simulink model "MMS_ESC_K_B_mixed_3"  (R2019b)
settings: Solver=ode4  StartTime=par.sym.TStart  StopTime=par.sym.TStop  FixedStep=par.sym.max_dt  MaxStep=par.sym.max_dt  RelTol=1e-3
undefined symbols (not defined in the file): b, B_0, beta_B, beta_K, eta_B, eta_K, k, K_0, k_B, k_K, lambda_B, lambda_K, m, m1_B0, m1_K0, m2_B0, m2_K0, N_delay, par, Q1_B0, Q1_K0, Q2_B0, Q2_K0, rho_B, rho_K, sigma, T_tran, W_B, W_K, w_wav
libraries: simulink x2
settings Model: Creator=Vitù  LastModifiedBy=User
settings DataIOCC: SaveFormat=Array  SaveOutput=off  SignalLogging=off  DSMLogging=off  ReturnWorkspaceOutputs=off  TimeSaveName=TIME  OutputSaveName=Yout  OutputOption=SpecifiedOutputTimes  OutputTimes=[par.sym.TStart:par.sym.Outputdt:par.sym.TStop]
settings OptimizationCC: ExpressionDepthLimit=2147483647  LifeSpan=inf
settings DebuggingCC: UnderspecifiedInitializationDetection=Classic  MergeDetectMultiDrivingBlocksExec=none  SolverPrmCheckMsg=warning  AllowSymbolicDim=off  StateNameClashWarn=warning  SFUnexpectedBacktrackingDiag=warning  SFNoUnconditionalDefaultTransitionDiag=warning  SFExecutionAtInitializationDiag=none  ArithmeticOperatorsInVariantConditions=warning
settings HardwareCC: ProdBitPerPointer=32  ProdBitPerSizeT=32  ProdBitPerPtrDiffT=32  ProdLargestAtomicFloat=None  ProdIntDivRoundTo=Undefined  ProdEndianess=Unspecified  ProdWordSize=32  ProdHWDeviceType=32-bit Generic
settings ModelReferenceCC: PropagateSignalLabelsOutOfModel=off
settings SFSimCC: SimUseLocalCustomCode=off  CustomCodeUndefinedFunction=UseInterfaceOnly
settings RTWCC: RTWUseLocalCustomCode=off
settings CodeAppCC: StateflowObjectComments=on
settings GRTTargetCC: TargetLangStandard=C89/C90 (ANSI)  GeneratePreprocessorConditionals=Disable all
settings ConfigComp: CovMetricSettings=dw  CovHtmlReporting=on  CovSaveCumulativeToWorkspaceVar=on  CovSaveSingleToWorkspaceVar=on  CovExternalEMLEnable=off  CovSFcnEnable=off
settings SimscapeCC: SimscapeNormalizeSystem=off
settings ConfigurationSet: Description=SimMechanics 2G

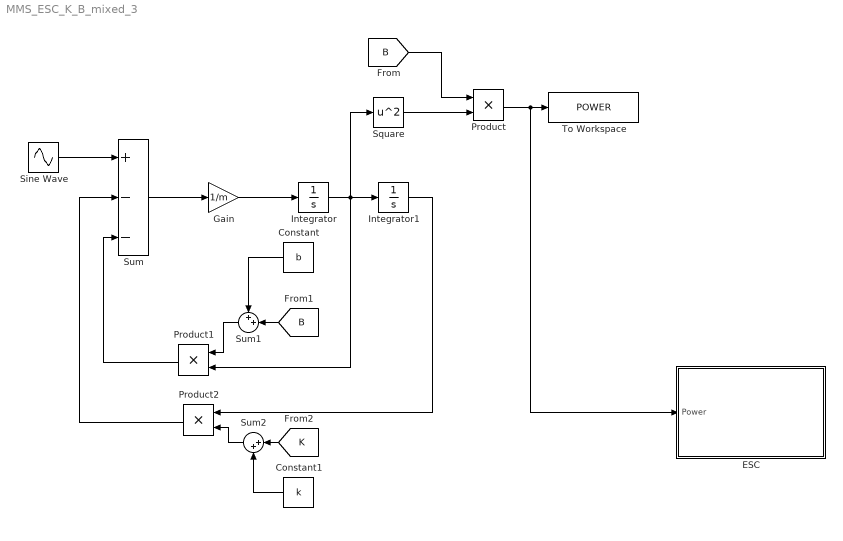
== system MMS_ESC_K_B_mixed_3 ==
  Constant : Constant  Value=b
  Constant1 : Constant  Value=k
  ESC : Subsystem
  Gain : Gain  Gain=1/m
  Integrator : Integrator
  Integrator1 : Integrator
  Product : Product
  Product1 : Product
  Product2 : Product
  Sine Wave : Sin  Amplitude=par.H  Frequency=w_wav  SampleTime=0
  Square : Math  Operator=square  SignedPower=off  SaturateOnIntegerOverflow=on
  Sum : Sum  Inputs=+--
  Sum1 : Sum  Inputs=++|
  Sum2 : Sum  Inputs=|++
  To Workspace : ToWorkspace  VariableName=POWER  SampleTime=-1
  wires:
  Integrator1/1 -> Product2/1
  Product/1 -> ESC/1(Power), To Workspace/1
  Product1/1 -> Sum/3
  Gain/1 -> Integrator/1
  Square/1 -> Product/2
  Sum/1 -> Gain/1
  Integrator/1 -> Product1/2, Square/1, Integrator1/1
  Product2/1 -> Sum/2
  Sine Wave/1 -> Sum/1
  [B] -> Product/1
  [B] -> Sum1/2
  Sum1/1 -> Product1/1
  Constant/1 -> Sum1/1
  [K] -> Sum2/1
  Sum2/1 -> Product2/2
  Constant1/1 -> Sum2/2

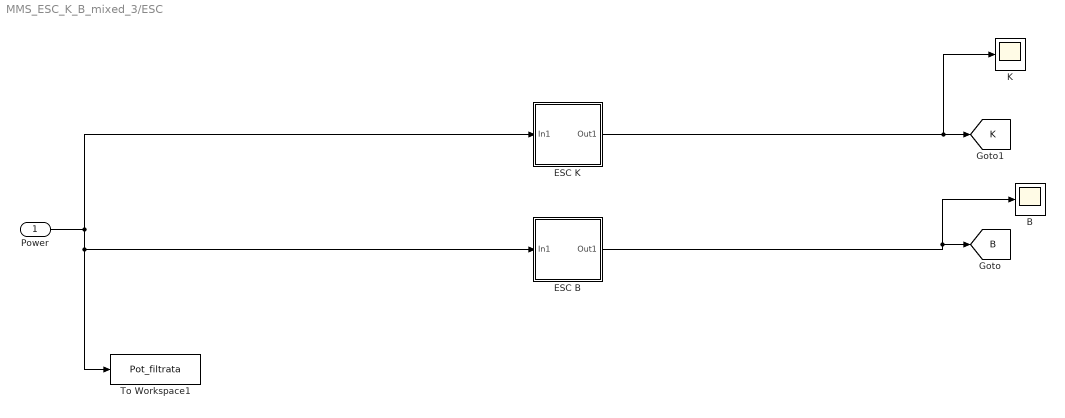
== system MMS_ESC_K_B_mixed_3/ESC ==
  Power : Inport
  B : Scope
  ESC B : Subsystem
  ESC K : Subsystem
  K : Scope
  To Workspace1 : ToWorkspace  VariableName=Pot_filtrata  SampleTime=-1
  tag scope: B=global, K=global
  wires:
  ESC B/1(Out1) -> B/1, [B]
  ESC K/1(Out1) -> K/1, [K]
  Power/1 -> To Workspace1/1, ESC B/1(In1), ESC K/1(In1)

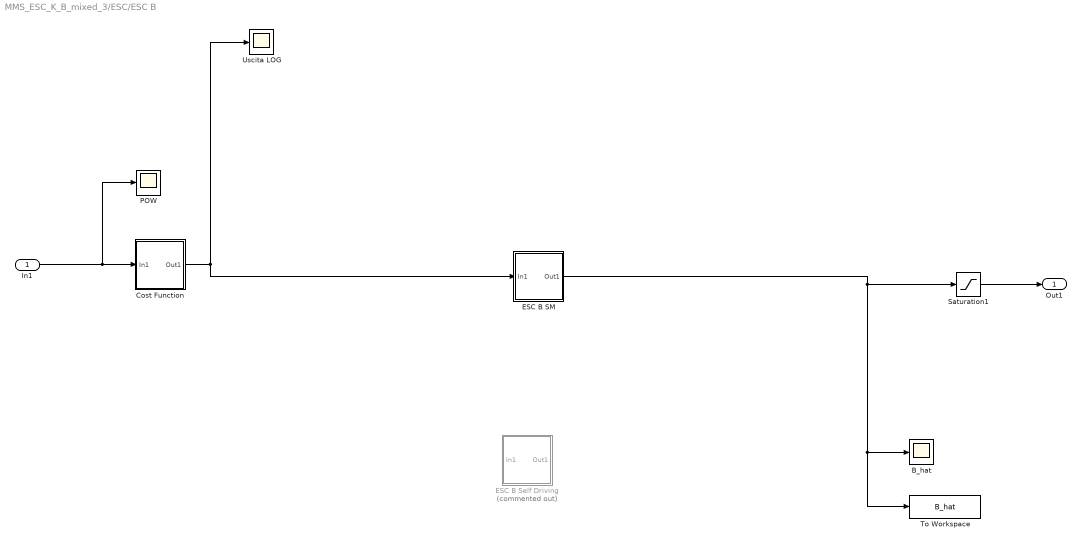
== system MMS_ESC_K_B_mixed_3/ESC/ESC B ==
  In1 : Inport
  B_hat : Scope
  Cost Function : Subsystem
  ESC B SM : Subsystem
  ESC B Self Driving : Subsystem  Commented=on
  POW : Scope
  Saturation1 : Saturate  UpperLimit=inf  LowerLimit=-b
  To Workspace : ToWorkspace  VariableName=B_hat  SampleTime=-1
  Uscita LOG : Scope
  Out1 : Outport
  wires:
  Cost Function/1(Out1) -> ESC B SM/1(In1), Uscita LOG/1
  In1/1 -> POW/1, Cost Function/1(In1)
  Saturation1/1 -> Out1/1
  ESC B SM/1(Out1) -> Saturation1/1, To Workspace/1, B_hat/1

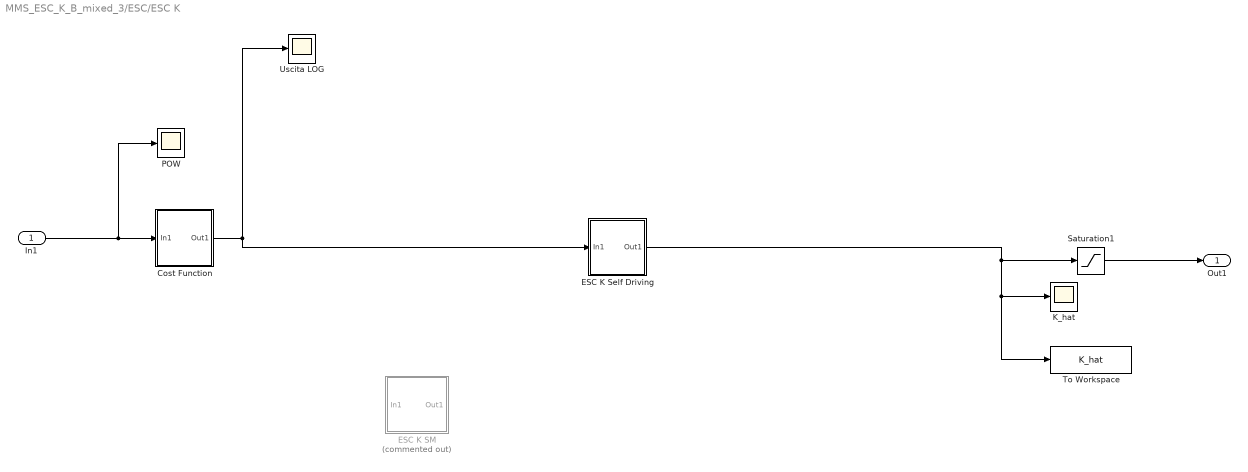
== system MMS_ESC_K_B_mixed_3/ESC/ESC K ==
  In1 : Inport
  Cost Function : Subsystem
  ESC K SM : Subsystem  Commented=on
  ESC K Self Driving : Subsystem
  K_hat : Scope
  POW : Scope
  Saturation1 : Saturate  UpperLimit=inf  LowerLimit=-k
  To Workspace : ToWorkspace  VariableName=K_hat  SampleTime=-1
  Uscita LOG : Scope
  Out1 : Outport
  wires:
  Cost Function/1(Out1) -> ESC K Self Driving/1(In1), Uscita LOG/1
  In1/1 -> POW/1, Cost Function/1(In1)
  Saturation1/1 -> Out1/1
  ESC K Self Driving/1(Out1) -> Saturation1/1, To Workspace/1, K_hat/1

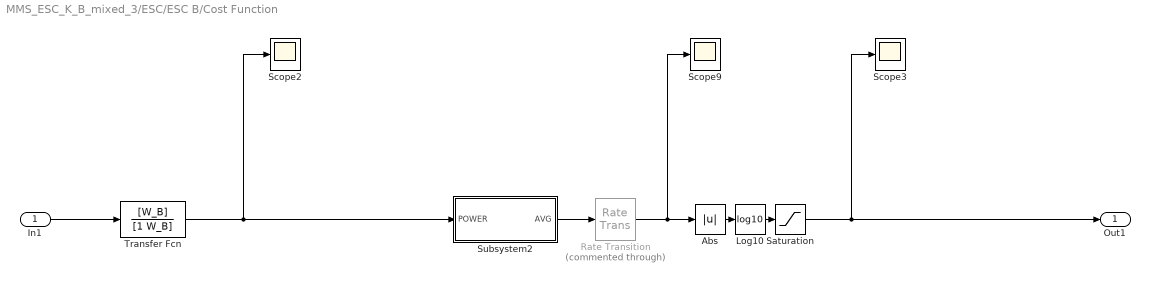
== system MMS_ESC_K_B_mixed_3/ESC/ESC B/Cost Function ==
  In1 : Inport
  Abs : Abs
  Log10 : Math  Operator=log10  SignedPower=off  SaturateOnIntegerOverflow=on
  Rate Transition : RateTransition  Commented=through
  Saturation : Saturate  UpperLimit=inf  LowerLimit=-40
  Scope2 : Scope
  Scope3 : Scope
  Scope9 : Scope
  Subsystem2 : Subsystem
  Transfer Fcn : TransferFcn  Numerator=[W_B]  Denominator=[1 W_B]
  Out1 : Outport
  wires:
  Subsystem2/1(AVG) -> Rate Transition/1
  Rate Transition/1 -> Abs/1, Scope9/1
  In1/1 -> Transfer Fcn/1
  Transfer Fcn/1 -> Subsystem2/1(POWER), Scope2/1
  Abs/1 -> Log10/1
  Log10/1 -> Saturation/1
  Saturation/1 -> Out1/1, Scope3/1

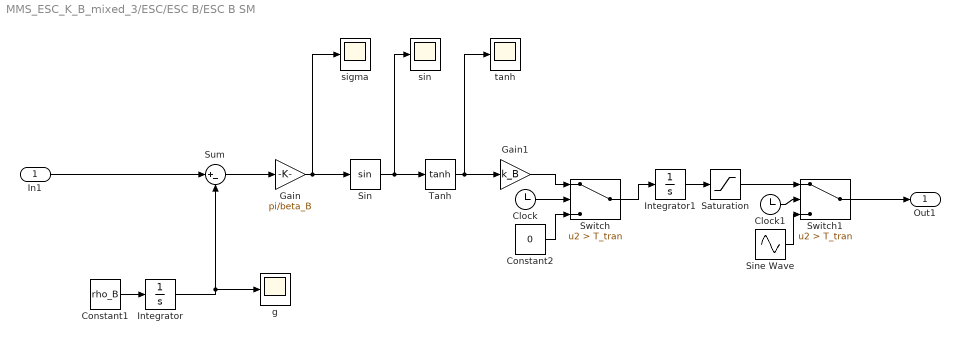
== system MMS_ESC_K_B_mixed_3/ESC/ESC B/ESC B SM ==
  In1 : Inport
  Clock : Clock
  Clock1 : Clock
  Constant1 : Constant  Value=rho_B
  Constant2 : Constant  Value=0
  Gain : Gain  Gain=pi/beta_B
  Gain1 : Gain  Gain=k_B
  Integrator : Integrator
  Integrator1 : Integrator  InitialCondition=B_0
  Saturation : Saturate  UpperLimit=inf  LowerLimit=5
  Sin : Trigonometry
  Sine Wave : Sin  Amplitude=5  Bias=B_0  Frequency=w_wav  SampleTime=0
  Sum : Sum  Inputs=|+-
  Switch : Switch  Criteria=u2 > Threshold  Threshold=T_tran
  Switch1 : Switch  Criteria=u2 > Threshold  Threshold=T_tran
  Tanh : Trigonometry  Operator=tanh
  g : Scope
  sigma : Scope
  sin : Scope
  tanh : Scope
  Out1 : Outport
  wires:
  Sin/1 -> sin/1, Tanh/1
  Constant1/1 -> Integrator/1
  Clock/1 -> Switch/2
  Integrator/1 -> g/1, Sum/2
  Sine Wave/1 -> Switch1/3
  In1/1 -> Sum/1
  Saturation/1 -> Switch1/1
  Gain/1 -> sigma/1, Sin/1
  Tanh/1 -> tanh/1, Gain1/1
  Clock1/1 -> Switch1/2
  Gain1/1 -> Switch/1
  Switch/1 -> Integrator1/1
  Sum/1 -> Gain/1
  Constant2/1 -> Switch/3
  Integrator1/1 -> Saturation/1
  Switch1/1 -> Out1/1

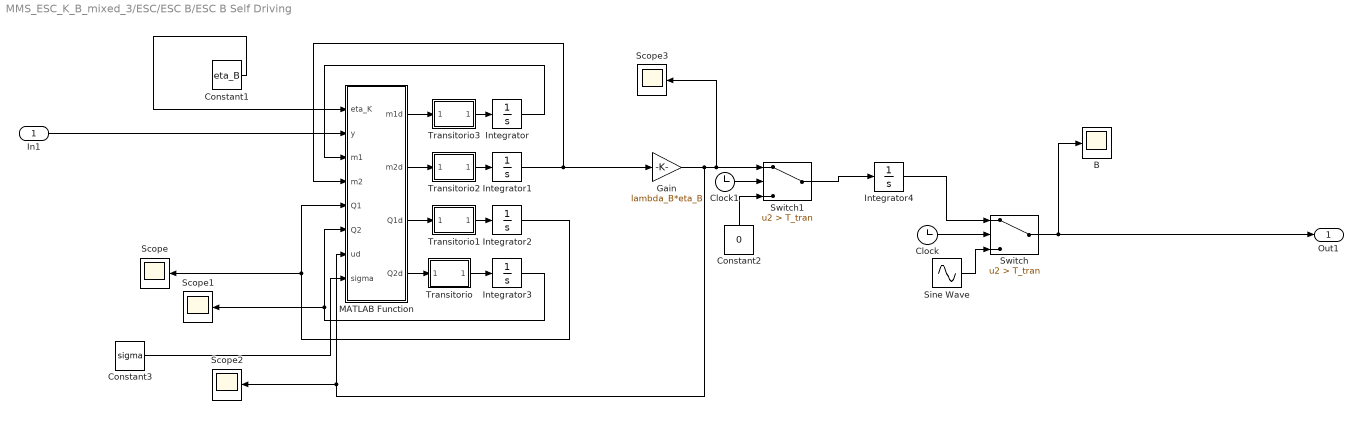
== system MMS_ESC_K_B_mixed_3/ESC/ESC B/ESC B Self Driving ==
  In1 : Inport
  B : Scope
  Clock : Clock
  Clock1 : Clock
  Constant1 : Constant  Value=eta_B
  Constant2 : Constant  Value=0
  Constant3 : Constant  Value=sigma
  Gain : Gain  Gain=lambda_B*eta_B
  Integrator : Integrator  InitialCondition=m1_B0
  Integrator1 : Integrator  InitialCondition=m2_B0
  Integrator2 : Integrator  InitialCondition=Q1_B0
  Integrator3 : Integrator  InitialCondition=Q2_B0
  Integrator4 : Integrator  InitialCondition=B_0
  MATLAB Function : MATLAB Function  TreatAsAtomicUnit=on
  Scope{,1..3} (4 alike) : Scope
  Sine Wave : Sin  Bias=B_0  SampleTime=0
  Switch : Switch  Criteria=u2 > Threshold  Threshold=T_tran
  Switch1 : Switch  Criteria=u2 > Threshold  Threshold=T_tran
  Transitorio : Subsystem
  Transitorio1 : Subsystem
  Transitorio2 : Subsystem
  Transitorio3 : Subsystem
  Out1 : Outport
  wires:
  Switch/1 -> Out1/1, B/1
  Integrator2/1 -> MATLAB Function/5(Q1), Scope/1
  Constant2/1 -> Switch1/3
  Gain/1 -> Scope3/1, Switch1/1, MATLAB Function/7(ud), Scope2/1
  Integrator1/1 -> Gain/1, MATLAB Function/4(m2)
  MATLAB Function/4(Q2d) -> Transitorio/1(In1)
  Integrator/1 -> MATLAB Function/3(m1)
  In1/1 -> MATLAB Function/2(y)
  Switch1/1 -> Integrator4/1
  MATLAB Function/1(m1d) -> Transitorio3/1(In1)
  Integrator3/1 -> MATLAB Function/6(Q2), Scope1/1
  Sine Wave/1 -> Switch/3
  MATLAB Function/2(m2d) -> Transitorio2/1(In1)
  Clock1/1 -> Switch1/2
  MATLAB Function/3(Q1d) -> Transitorio1/1(In1)
  Constant1/1 -> MATLAB Function/1(eta_K)
  Constant3/1 -> MATLAB Function/8(sigma)
  Integrator4/1 -> Switch/1
  Clock/1 -> Switch/2
  Transitorio/1(Out1) -> Integrator3/1
  Transitorio1/1(Out1) -> Integrator2/1
  Transitorio2/1(Out1) -> Integrator1/1
  Transitorio3/1(Out1) -> Integrator/1

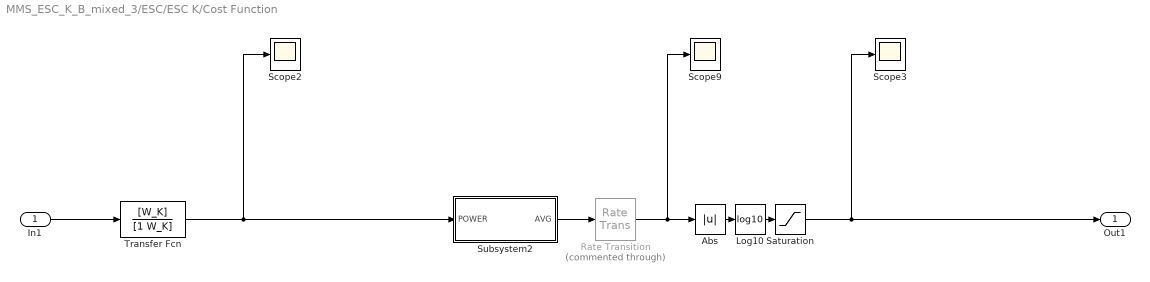
== system MMS_ESC_K_B_mixed_3/ESC/ESC K/Cost Function ==
  In1 : Inport
  Abs : Abs
  Log10 : Math  Operator=log10  SignedPower=off  SaturateOnIntegerOverflow=on
  Rate Transition : RateTransition  Commented=through
  Saturation : Saturate  UpperLimit=inf  LowerLimit=-40
  Scope2 : Scope
  Scope3 : Scope
  Scope9 : Scope
  Subsystem2 : Subsystem
  Transfer Fcn : TransferFcn  Numerator=[W_K]  Denominator=[1 W_K]
  Out1 : Outport
  wires:
  Subsystem2/1(AVG) -> Rate Transition/1
  Rate Transition/1 -> Abs/1, Scope9/1
  In1/1 -> Transfer Fcn/1
  Transfer Fcn/1 -> Subsystem2/1(POWER), Scope2/1
  Abs/1 -> Log10/1
  Log10/1 -> Saturation/1
  Saturation/1 -> Out1/1, Scope3/1

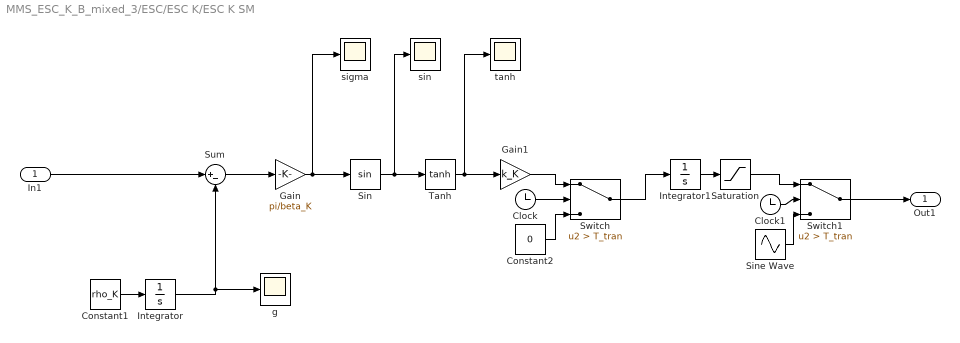
== system MMS_ESC_K_B_mixed_3/ESC/ESC K/ESC K SM ==
  In1 : Inport
  Clock : Clock
  Clock1 : Clock
  Constant1 : Constant  Value=rho_K
  Constant2 : Constant  Value=0
  Gain : Gain  Gain=pi/beta_K
  Gain1 : Gain  Gain=k_K
  Integrator : Integrator
  Integrator1 : Integrator  InitialCondition=K_0
  Saturation : Saturate  UpperLimit=inf  LowerLimit=100
  Sin : Trigonometry
  Sine Wave : Sin  Amplitude=50  Bias=K_0  Frequency=w_wav  SampleTime=0
  Sum : Sum  Inputs=|+-
  Switch : Switch  Criteria=u2 > Threshold  Threshold=T_tran
  Switch1 : Switch  Criteria=u2 > Threshold  Threshold=T_tran
  Tanh : Trigonometry  Operator=tanh
  g : Scope
  sigma : Scope
  sin : Scope
  tanh : Scope
  Out1 : Outport
  wires:
  Sum/1 -> Gain/1
  Tanh/1 -> tanh/1, Gain1/1
  Integrator/1 -> g/1, Sum/2
  Gain/1 -> sigma/1, Sin/1
  Switch/1 -> Integrator1/1
  Gain1/1 -> Switch/1
  Sine Wave/1 -> Switch1/3
  Sin/1 -> sin/1, Tanh/1
  Constant1/1 -> Integrator/1
  Constant2/1 -> Switch/3
  Switch1/1 -> Out1/1
  Clock1/1 -> Switch1/2
  Integrator1/1 -> Saturation/1
  Saturation/1 -> Switch1/1
  Clock/1 -> Switch/2
  In1/1 -> Sum/1

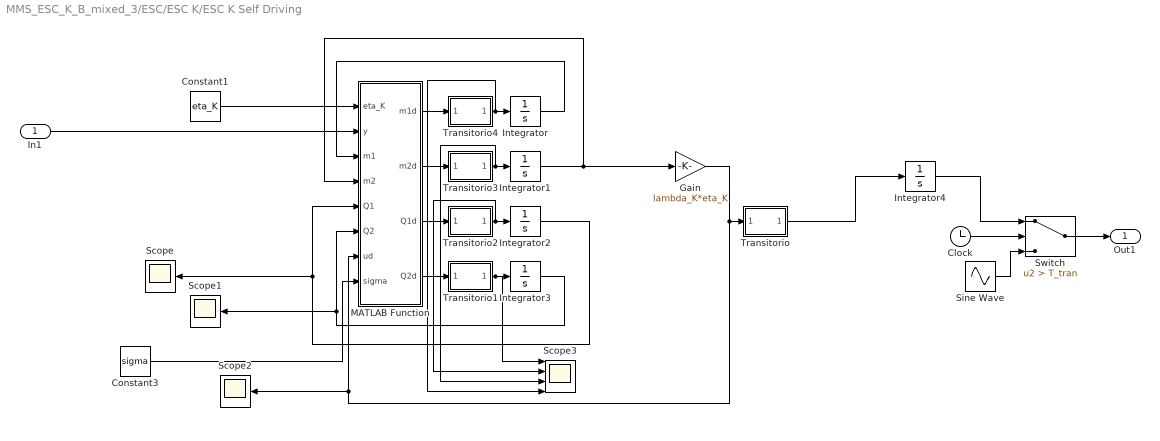
== system MMS_ESC_K_B_mixed_3/ESC/ESC K/ESC K Self Driving ==
  In1 : Inport
  Clock : Clock
  Constant1 : Constant  Value=eta_K
  Constant3 : Constant  Value=sigma
  Gain : Gain  Gain=lambda_K*eta_K
  Integrator : Integrator  InitialCondition=m1_K0
  Integrator1 : Integrator  InitialCondition=m2_K0
  Integrator2 : Integrator  InitialCondition=Q1_K0
  Integrator3 : Integrator  InitialCondition=Q2_K0
  Integrator4 : Integrator  InitialCondition=K_0
  MATLAB Function : MATLAB Function  TreatAsAtomicUnit=on
  Scope : Scope
  Scope1 : Scope
  Scope2 : Scope
  Scope3 : Scope  NumInputPorts=4
  Sine Wave : Sin  Bias=K_0  SampleTime=0
  Switch : Switch  Criteria=u2 > Threshold  Threshold=T_tran
  Transitorio : Subsystem
  Transitorio1 : Subsystem
  Transitorio2 : Subsystem
  Transitorio3 : Subsystem
  Transitorio4 : Subsystem
  Out1 : Outport
  wires:
  Sine Wave/1 -> Switch/3
  Gain/1 -> Transitorio/1(In1), MATLAB Function/7(ud), Scope2/1
  Constant1/1 -> MATLAB Function/1(eta_K)
  Integrator1/1 -> Gain/1, MATLAB Function/4(m2)
  Integrator3/1 -> MATLAB Function/6(Q2), Scope1/1
  Integrator4/1 -> Switch/1
  Constant3/1 -> MATLAB Function/8(sigma)
  MATLAB Function/1(m1d) -> Transitorio4/1(In1)
  MATLAB Function/2(m2d) -> Transitorio3/1(In1)
  MATLAB Function/3(Q1d) -> Transitorio2/1(In1)
  Integrator/1 -> MATLAB Function/3(m1)
  MATLAB Function/4(Q2d) -> Transitorio1/1(In1)
  Clock/1 -> Switch/2
  Integrator2/1 -> MATLAB Function/5(Q1), Scope/1
  Switch/1 -> Out1/1
  In1/1 -> MATLAB Function/2(y)
  Transitorio/1(Out1) -> Integrator4/1
  Transitorio1/1(Out1) -> Scope3/1, Integrator3/1
  Transitorio2/1(Out1) -> Scope3/2, Integrator2/1
  Transitorio3/1(Out1) -> Scope3/3, Integrator1/1
  Transitorio4/1(Out1) -> Scope3/4, Integrator/1

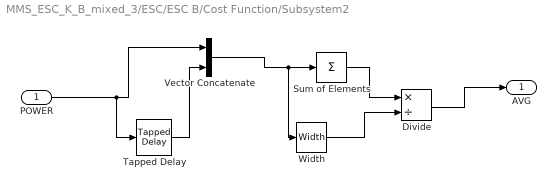
== system MMS_ESC_K_B_mixed_3/ESC/ESC B/Cost Function/Subsystem2 ==
  POWER : Inport
  Divide : Product  Inputs=*/
  Sum of Elements : Sum  Inputs=+
  Tapped Delay : simulink/Discrete/Tapped Delay  vinit=0  samptime=-1  NumDelays=N_delay  DelayOrder=Oldest  includeCurrent=off
  Vector Concatenate : Concatenate
  Width : Width
  AVG : Outport
  wires:
  POWER/1 -> Tapped Delay/1, Vector Concatenate/1
  Tapped Delay/1 -> Vector Concatenate/2
  Vector Concatenate/1 -> Width/1, Sum of Elements/1
  Sum of Elements/1 -> Divide/1
  Width/1 -> Divide/2
  Divide/1 -> AVG/1

== system MMS_ESC_K_B_mixed_3/ESC/ESC B/ESC B Self Driving/Transitorio ==
  In1 : Inport
  Clock1 : Clock
  Constant2 : Constant  Value=0
  Switch1 : Switch  Criteria=u2 > Threshold  Threshold=T_tran
  Out1 : Outport
  wires:
  Constant2/1 -> Switch1/3
  Switch1/1 -> Out1/1
  Clock1/1 -> Switch1/2
  In1/1 -> Switch1/1

== system MMS_ESC_K_B_mixed_3/ESC/ESC B/ESC B Self Driving/Transitorio1 ==
  In1 : Inport
  Clock1 : Clock
  Constant2 : Constant  Value=0
  Switch1 : Switch  Criteria=u2 > Threshold  Threshold=T_tran
  Out1 : Outport
  wires:
  Constant2/1 -> Switch1/3
  Switch1/1 -> Out1/1
  Clock1/1 -> Switch1/2
  In1/1 -> Switch1/1

== system MMS_ESC_K_B_mixed_3/ESC/ESC B/ESC B Self Driving/Transitorio2 ==
  In1 : Inport
  Clock1 : Clock
  Constant2 : Constant  Value=0
  Switch1 : Switch  Criteria=u2 > Threshold  Threshold=T_tran
  Out1 : Outport
  wires:
  Constant2/1 -> Switch1/3
  Switch1/1 -> Out1/1
  Clock1/1 -> Switch1/2
  In1/1 -> Switch1/1

== system MMS_ESC_K_B_mixed_3/ESC/ESC B/ESC B Self Driving/Transitorio3 ==
  In1 : Inport
  Clock1 : Clock
  Constant2 : Constant  Value=0
  Switch1 : Switch  Criteria=u2 > Threshold  Threshold=T_tran
  Out1 : Outport
  wires:
  Constant2/1 -> Switch1/3
  Switch1/1 -> Out1/1
  Clock1/1 -> Switch1/2
  In1/1 -> Switch1/1

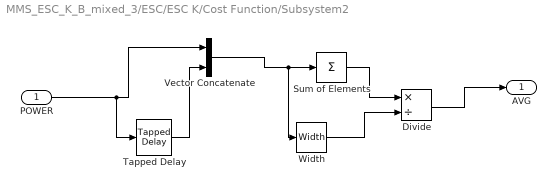
== system MMS_ESC_K_B_mixed_3/ESC/ESC K/Cost Function/Subsystem2 ==
  POWER : Inport
  Divide : Product  Inputs=*/
  Sum of Elements : Sum  Inputs=+
  Tapped Delay : simulink/Discrete/Tapped Delay  vinit=0  samptime=-1  NumDelays=N_delay  DelayOrder=Oldest  includeCurrent=off
  Vector Concatenate : Concatenate
  Width : Width
  AVG : Outport
  wires:
  POWER/1 -> Tapped Delay/1, Vector Concatenate/1
  Tapped Delay/1 -> Vector Concatenate/2
  Vector Concatenate/1 -> Width/1, Sum of Elements/1
  Sum of Elements/1 -> Divide/1
  Width/1 -> Divide/2
  Divide/1 -> AVG/1

== system MMS_ESC_K_B_mixed_3/ESC/ESC K/ESC K Self Driving/Transitorio ==
  In1 : Inport
  Clock1 : Clock
  Constant2 : Constant  Value=0
  Switch1 : Switch  Criteria=u2 > Threshold  Threshold=T_tran
  Out1 : Outport
  wires:
  Constant2/1 -> Switch1/3
  Switch1/1 -> Out1/1
  Clock1/1 -> Switch1/2
  In1/1 -> Switch1/1

== system MMS_ESC_K_B_mixed_3/ESC/ESC K/ESC K Self Driving/Transitorio1 ==
  In1 : Inport
  Clock1 : Clock
  Constant2 : Constant  Value=0
  Switch1 : Switch  Criteria=u2 > Threshold  Threshold=T_tran
  Out1 : Outport
  wires:
  Constant2/1 -> Switch1/3
  Switch1/1 -> Out1/1
  Clock1/1 -> Switch1/2
  In1/1 -> Switch1/1

== system MMS_ESC_K_B_mixed_3/ESC/ESC K/ESC K Self Driving/Transitorio2 ==
  In1 : Inport
  Clock1 : Clock
  Constant2 : Constant  Value=0
  Switch1 : Switch  Criteria=u2 > Threshold  Threshold=T_tran
  Out1 : Outport
  wires:
  Constant2/1 -> Switch1/3
  Switch1/1 -> Out1/1
  Clock1/1 -> Switch1/2
  In1/1 -> Switch1/1

== system MMS_ESC_K_B_mixed_3/ESC/ESC K/ESC K Self Driving/Transitorio3 ==
  In1 : Inport
  Clock1 : Clock
  Constant2 : Constant  Value=0
  Switch1 : Switch  Criteria=u2 > Threshold  Threshold=T_tran
  Out1 : Outport
  wires:
  Constant2/1 -> Switch1/3
  Switch1/1 -> Out1/1
  Clock1/1 -> Switch1/2
  In1/1 -> Switch1/1

== system MMS_ESC_K_B_mixed_3/ESC/ESC K/ESC K Self Driving/Transitorio4 ==
  In1 : Inport
  Clock1 : Clock
  Constant2 : Constant  Value=0
  Switch1 : Switch  Criteria=u2 > Threshold  Threshold=T_tran
  Out1 : Outport
  wires:
  Constant2/1 -> Switch1/3
  Switch1/1 -> Out1/1
  Clock1/1 -> Switch1/2
  In1/1 -> Switch1/1

== matlab function MMS_ESC_K_B_mixed_3/ESC/ESC K/ESC K Self Driving/MATLAB Function ==
  data: eta_K input; m1d output; y input; m1 input; m2 input; Q1 input; Q2 input; ud input; m2d output; Q1d output; Q2d output; sigma input
function [m1d,m2d,Q1d,Q2d] = SDK(eta_K,y,m1,m2,Q1,Q2,ud,sigma)
m1d = eta_K*(y-m1);
m2d = eta_K*Q1*Q2*(y-m1-Q1*m2)-sigma*eta_K*Q2*m2;
Q1d = -eta_K*Q1 + ud;
Q2d = eta_K*Q2 -eta_K*(Q1*Q2)^2-sigma*eta_K*Q2^2;

== matlab function MMS_ESC_K_B_mixed_3/ESC/ESC B/ESC B Self Driving/MATLAB Function ==
  data: eta_K input; m1d output; y input; m1 input; m2 input; Q1 input; Q2 input; ud input; m2d output; Q1d output; Q2d output; sigma input
function [m1d,m2d,Q1d,Q2d] = SDK(eta_K,y,m1,m2,Q1,Q2,ud,sigma)
m1d = eta_K*(y-m1);
m2d = eta_K*Q1*Q2*(y-m1-Q1*m2)-sigma*eta_K*Q2*m2;
Q1d = -eta_K*Q1 + ud;
Q2d = eta_K*Q2 -eta_K*(Q1*Q2)^2-sigma*eta_K*Q2^2;
